simulink model "tetra"  (R2016a)
settings: Solver=VariableStepAuto  StartTime=0.0  StopTime=2  RelTol=1e-3
libraries: aausat3_lib x1
settings Model: Creator=jn  LastModifiedBy=jn
settings DataIOCC: LimitDataPoints=on
settings DebuggingCC: AllowSymbolicDim=off
settings ModelReferenceCC: PropagateSignalLabelsOutOfModel=off
settings GRTTargetCC: GeneratePreprocessorConditionals=Use local settings

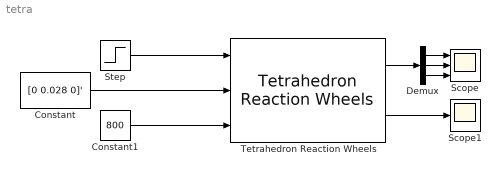
== system tetra ==
  Constant : Constant  Value=[0 0.028 0]'  VectorParams1D=off
  Constant1 : Constant  Value=800
  Demux : Demux  Outputs=3
  Scope : Scope  NumInputPorts=3
  Scope1 : Scope
  Step : Step  Before=[1.5 1.5 1.5 1.5]'  After=[1 1 1 2]'  SampleTime=0  VectorParams1D=off
  Tetrahedron Reaction Wheels : aausat3_lib/Actuator Emulation/Tetrahedron Reaction Wheels  q_S_Tetra=[0 0 1 0]  I_w=diag([0.148 0.148 0.0435])*10e-6  coriolis_on=on
  wires:
  Tetrahedron Reaction Wheels/1 -> Demux/1
  Demux/1 -> Scope/1
  Demux/2 -> Scope/2
  Demux/3 -> Scope/3
  Tetrahedron Reaction Wheels/2 -> Scope1/1
  Constant/1 -> Tetrahedron Reaction Wheels/2
  Constant1/1 -> Tetrahedron Reaction Wheels/3
  Step/1 -> Tetrahedron Reaction Wheels/1
